simulink model "demoCV"  (R2018b)
settings: Solver=VariableStepAuto  StartTime=0.0  StopTime=100  RelTol=1e-3
undefined symbols (not defined in the file or in its folder): gray
libraries: visionstatistics x1, visiontextngfix x1, dspvision x1, imaqlib x1
settings Model: Creator=User  LastModifiedBy=User

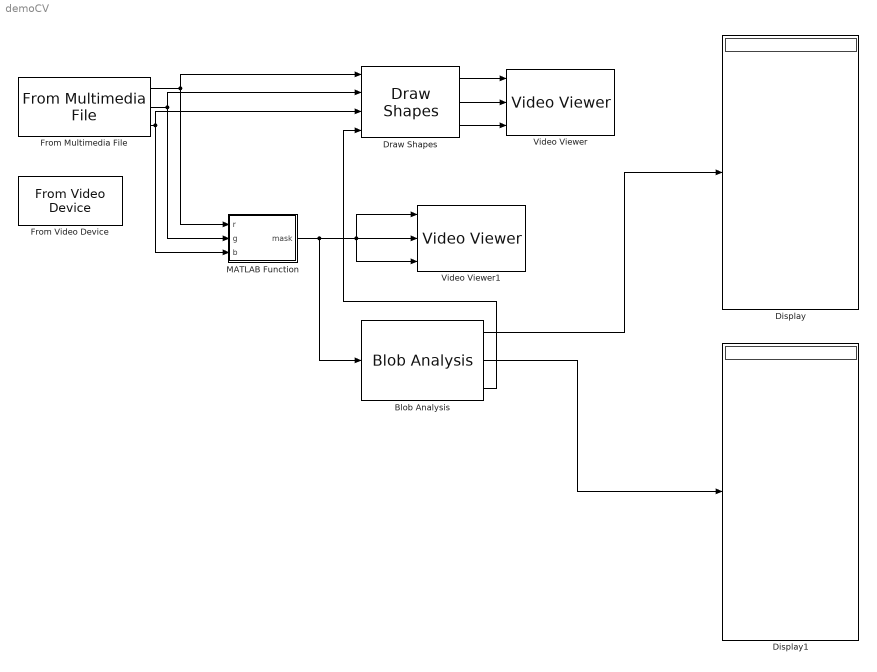
== system demoCV ==
  Blob Analysis : visionstatistics/Blob Analysis  Tag=vipblks_row_conv  area=on  centroid=on  bBox=on  majorAxis=off  minorAxis=off  angle=off  eccentricity=off  equivDiameterSq=off  extent=off  perimeter=off  maxBlobs=50  warnIfNumBlobsExceeded=on  isCount=off  useMinArea=off  minArea=0  useMaxArea=off  maxArea=intmax('uint32')  excludeBorderBlob=off  outDT=double  isOutVarDim=off  isFill=on  fillValues=-1  conn=8  isLabel=off  outputMode=Binary point scaling  outputWordLength=32  outputFracLength=16  firstCoeffMode=Binary point scaling  firstCoeffWordLength=16  firstCoeffFracLength=14  secondCoeffMode=Binary point scaling  secondCoeffWordLength=32  secondCoeffFracLength=16  accumMode=Binary point scaling  accumWordLength=32  accumFracLength=0  prodOutputMode=Binary point scaling  prodOutputWordLength=32  prodOutputFracLength=16  roundingMode=Floor  overflowMode=off
      settings: SourceProductName=Computer Vision System Toolbox
  Display : Display
  Display1 : Display
  Draw Shapes : visiontextngfix/Draw Shapes  shape=Rectangles  fill=off  lineWidth=1  fillClrSource=Specify via dialog  display=User-specified value  intensity=200  color=[255 0 0]  opacity=0.6  viewport=Entire image  antialiasing=off  inType=Obsolete  imagePorts=Separate color signals  prodOutputMode=Binary point scaling  prodOutputWordLength=32  prodOutputFracLength=14  memoryMode=Specify word length  memoryWordLength=16  memoryFracLength=15  roundingMode=Floor  overflowMode=off
      settings: SourceProductName=Computer Vision System Toolbox
  From Multimedia File : dspvision/From Multimedia File  inputFilename=C:\Program Files\MATLAB\R2018b\toolbox\vision\visiondata\vipscenevideoclip.avi  loop=on  numPlays=inf  outputStreams=Video only  videoDataType=uint8  audioDataType=int16  inheritSampleTime=on  userDefinedSampleTime=1/30  noAudioOutput=off  isIntensityVideo=off  fourcc=RGB  colorVideoFormat=Separate color signals  outputEOF=off  dataOrg=Column-major  audioFrameSize=1024  computeAudioFrameSize=off  outSamplingMode=Sample based
      settings: SourceProductBaseCode=VP
  From Video Device : imaqlib/From Video Device  DeviceMenu=(none)  Device=(none)  ObjConstructor=(none)  VideoFormatMenu=(none)  VideoFormat=(none)  VideoSource=none  ROIPosition=(none)  EnableHWTrigger=off  TriggerConfiguration=(none)  SampleTime=1/30  OutputPortsMode=One multidimensional signal  DataType=single  CanDoHWTrigger=no  ReturnedColorSpace=rgb  BlockHandle=6.0001  ROIWidth=100  ROIHeight=100  ROIColumn=0  ROIRow=0  EngXMLPath=C:\Program Files\MATLAB\R2018b\toolbox\imaq\imaq\private  DevXMLPath=/mathworks/devel/bat/BR2018bd/build/matlab/toolbox/imaq/imaqadaptors/glnxa64/mwdemoimaq.so  EngLibPath=C:\Program Files\MATLAB\R2018b\toolbox\imaq\imaqblks\imaqmex\win64  ColorSpace=rgb  BayerSensorAlignment=grbg
      settings: SourceProductName=Image Acquisition Toolbox
  MATLAB Function : MATLAB Function  TreatAsAtomicUnit=on
  Video Viewer : VideoViewer  imagePorts=separate color signals  colormapValue=gray(256)  FigPos=[559 583 418 304]
  Video Viewer1 : VideoViewer  imagePorts=separate color signals  FigPos=[983.4 581.2 417.6 304]
  wires:
  From Multimedia File/1 -> Draw Shapes/1, MATLAB Function/1(r)
  From Multimedia File/2 -> Draw Shapes/2, MATLAB Function/2(g)
  From Multimedia File/3 -> Draw Shapes/3, MATLAB Function/3(b)
  MATLAB Function/1(mask) -> Blob Analysis/1, Video Viewer1/3, Video Viewer1/2, Video Viewer1/1
  Blob Analysis/1 -> Display/1
  Blob Analysis/2 -> Display1/1
  Blob Analysis/3 -> Draw Shapes/4
  Draw Shapes/1 -> Video Viewer/1
  Draw Shapes/2 -> Video Viewer/2
  Draw Shapes/3 -> Video Viewer/3

== matlab function demoCV/MATLAB Function ==
  data: r input; mask output; g input; b input
function mask = fcn(r,g,b)


Gmin=200;
mask1=Gmin<g;
mask2=b<(g-20);
mask3=r<(g-1);


mask = (mask1&mask2&mask3);
